simulink model "signals"  (R2023a)
settings: Solver=VariableStepAuto  StartTime=0.0  StopTime=10.0  RelTol=1e-3
settings Model: Creator=u29w13  LastModifiedBy=u29w13

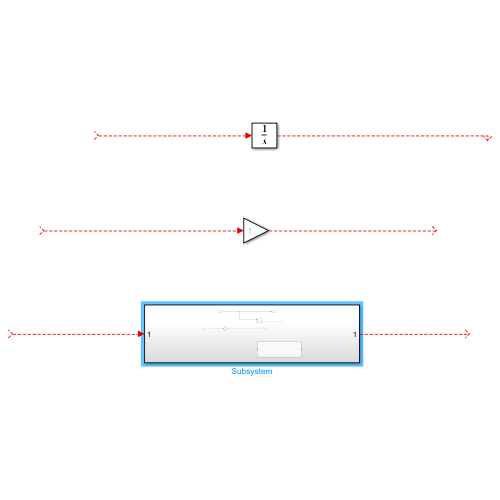
[thumbnail: Simulink's stored preview of the top-level diagram]
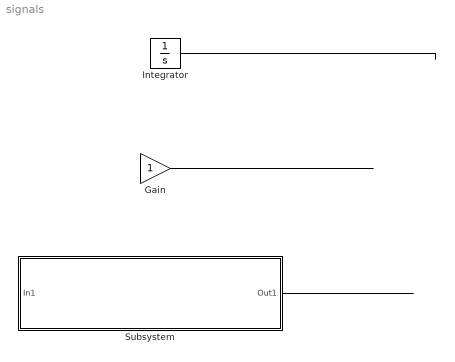
== system signals ==
  Gain : Gain
  Integrator : Integrator
  Subsystem : Subsystem
  wires:
  ? -> Integrator/1
  Integrator/1 -> ?
  Gain/1 -> ?
  ? -> Gain/1
  ? -> Subsystem/1(In1)
  Subsystem/1(Out1) -> ?

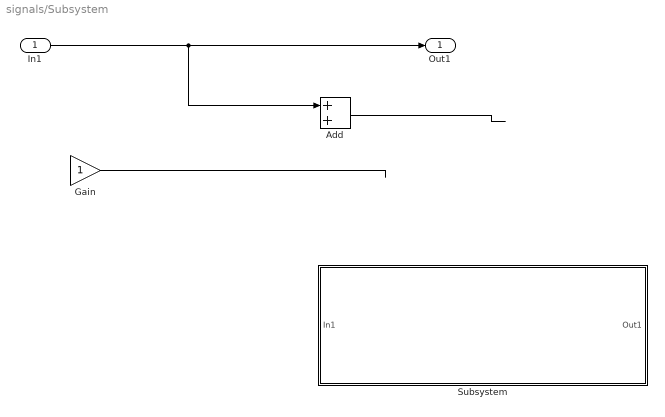
== system signals/Subsystem ==
  In1 : Inport
  Add : Sum
  Gain : Gain
  Subsystem : Subsystem
  Out1 : Outport
  wires:
  In1/1 -> Add/1, Out1/1
  Gain/1 -> ?
  ? -> Gain/1
  Add/1 -> ?

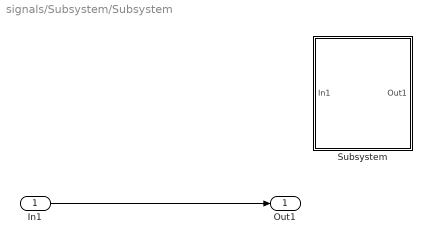
== system signals/Subsystem/Subsystem ==
  In1 : Inport
  Subsystem : Subsystem
  Out1 : Outport
  wires:
  In1/1 -> Out1/1

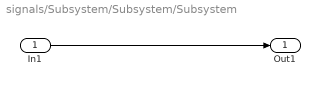
== system signals/Subsystem/Subsystem/Subsystem ==
  In1 : Inport
  Out1 : Outport
  wires:
  In1/1 -> Out1/1
